simulink model "geometric_control_ceil_ground"  (R2025a)
settings: Solver=VariableStepAuto  StartTime=0.0  StopTime=t_total(end)  RelTol=1e-3
StopFcn:
  | autoplot;
values from neighbouring files (symbols this model uses):
  Ib = diag([params.Ix, params.Iy, params.Iz])    [setup_mission.m]
  lin_vel_0 = [0; 0; 0]    [setup_mission.m]
  mass = params.m    [setup_mission.m]
  pos_0 = p_ref(:,1) + offset_init    [setup_mission.m]
  Ts = dt    (= 0.001)    [setup_mission.m]
  w_bb_0 = [0; 0; 0]    [setup_mission.m]
undefined symbols (not defined in the file or in its folder): dspblkCoreblockFVToolHelper, gcbh
libraries: robotcorelib x2, uavutilslib x1
settings Model: Creator=fabioruggiero  LastModifiedBy=marco
settings ModelReferenceCC: EnableRefExpFcnMdlSchedulingChecks=on
settings RTWCC: GPUComputeCapability=3.5

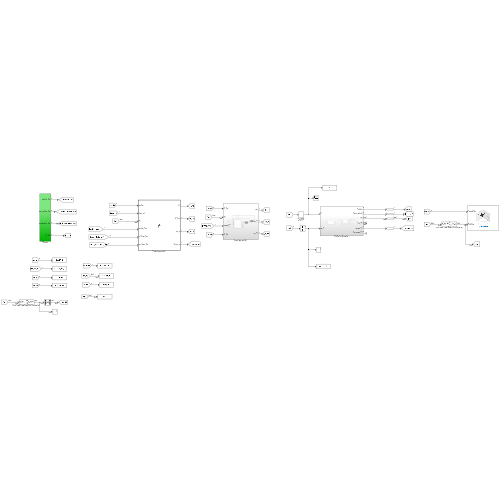
[thumbnail: Simulink's stored preview of the top-level diagram]
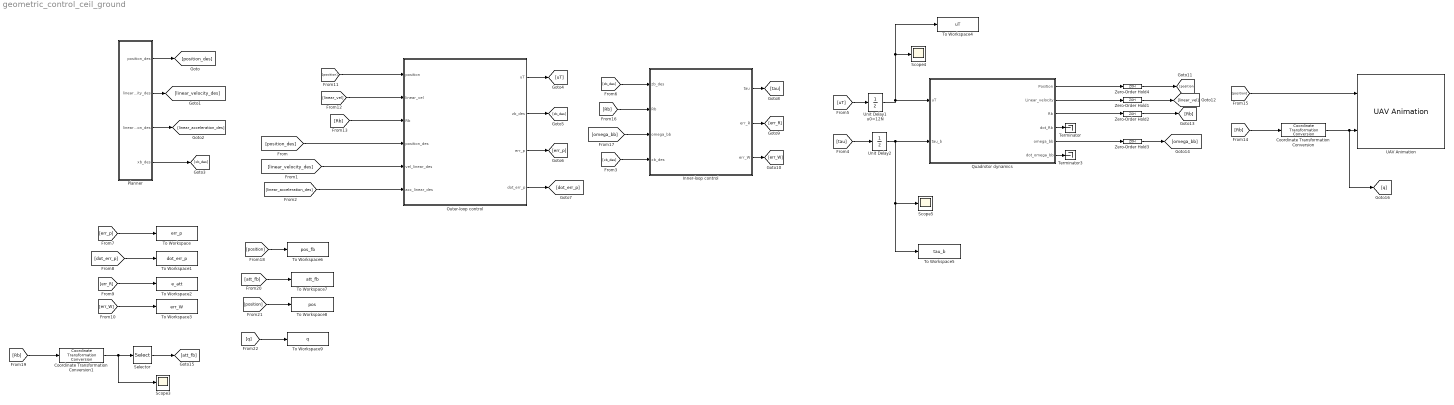
== system geometric_control_ceil_ground ==
  Coordinate Transformation Conversion : robotcorelib/Coordinate Transformation Conversion  InputRepresentation=Rotation Matrix  InputEulerSequence=ZYX  ShowTrVecInputPort=on  OutputRepresentation=Quaternion  OutputEulerSequence=ZYX  ShowTrVecOutputPort=on  SimulateUsing=Interpreted execution
  Coordinate Transformation Conversion1 : robotcorelib/Coordinate Transformation Conversion  InputRepresentation=Rotation Matrix  InputEulerSequence=ZYX  ShowTrVecInputPort=on  OutputRepresentation=Euler Angles  OutputEulerSequence=ZYX  ShowTrVecOutputPort=on  SimulateUsing=Interpreted execution
  Inner-loop control : Subsystem
  Outer-loop control : MATLAB Function  TreatAsAtomicUnit=on
  Planner : Subsystem
  Quadrotor dynamics : Subsystem
  Scope3 : Scope
      settings: ActiveDisplayYMinimum=-1  ActiveDisplayYMaximum=1  DataLoggingVariableName=ScopeData3
  Scope4 : Scope
      settings: ActiveDisplayYMinimum=-1  ActiveDisplayYMaximum=1  DataLoggingVariableName=ScopeData4
  Scope5 : Scope
      settings: ActiveDisplayYMinimum=-1  ActiveDisplayYMaximum=1  DataLoggingVariableName=ScopeData5
  Selector : Selector  InputPortWidth=3  IndexOptions=Index vector (dialog)  Indices=[3, 2, 1]  OutputSizes=1
  Terminator : Terminator
  Terminator3 : Terminator
  To Workspace : ToWorkspace  VariableName=err_p  SaveFormat=Timeseries  SampleTime=Ts
  To Workspace1 : ToWorkspace  VariableName=dot_err_p  SaveFormat=Timeseries  SampleTime=Ts
  To Workspace2 : ToWorkspace  VariableName=e_att  SaveFormat=Timeseries  SampleTime=-1
  To Workspace3 : ToWorkspace  VariableName=err_W  SaveFormat=Timeseries  SampleTime=-1
  To Workspace4 : ToWorkspace  VariableName=uT  SaveFormat=Timeseries  SampleTime=-1
  To Workspace5 : ToWorkspace  VariableName=tau_b  SaveFormat=Timeseries  SampleTime=-1
  To Workspace6 : ToWorkspace  VariableName=pos_fb  SaveFormat=Timeseries  SampleTime=-1
  To Workspace7 : ToWorkspace  VariableName=att_fb  SaveFormat=Timeseries  SampleTime=-1
  To Workspace8 : ToWorkspace  VariableName=pos  SaveFormat=Timeseries  SampleTime=-1
  To Workspace9 : ToWorkspace  VariableName=q  SaveFormat=Timeseries  SampleTime=-1
  UAV Animation : uavutilslib/UAV Animation  NumUAV=1  DynamicUAVConfig=off  UAVType=Multirotor  UAVSize=1  UAVColor=[1 0 0]  UAVTrajectoryAlpha=1  InertialZDirection=Down  RotationFormat=Quaternion  DrawMarkers=off  SampleTime=0.01
  Unit Delay1 u0=12N : UnitDelay  InitialCondition=12  SampleTime=Ts
  Unit Delay2 : UnitDelay  InitialCondition=[0 0 0]  SampleTime=Ts
  Zero-Order Hold{1..4} (4 alike) : ZeroOrderHold  SampleTime=Ts
  wires:
  Unit Delay1 u0=12N/1 -> Quadrotor dynamics/1(uT), To Workspace4/1, Scope4/1
  Quadrotor dynamics/1(Position) -> Zero-Order Hold4/1
  Quadrotor dynamics/2(Linear_velocity) -> Zero-Order Hold1/1
  Quadrotor dynamics/3(Rb) -> Zero-Order Hold2/1
  Quadrotor dynamics/5(omega_bb) -> Zero-Order Hold3/1
  Unit Delay2/1 -> Quadrotor dynamics/2(tau_b), Scope5/1, To Workspace5/1
  Quadrotor dynamics/4(dot_Rb) -> Terminator/1
  Quadrotor dynamics/6(dot_omega_bb) -> Terminator3/1
  Coordinate Transformation Conversion/1 -> [q], UAV Animation/2
  Inner-loop control/2(err_R) -> [err_R]
  Inner-loop control/3(err_W) -> [err_W]
  Planner/1(position_des) -> [position_des]
  Planner/2(linear_velocity_des) -> [linear_velocity_des]
  Planner/3(linear_acceleration_des) -> [linear_acceleration_des]
  Planner/4(xb_des) -> [xb_des]
  [position_des] -> Outer-loop control/4(position_des)
  [linear_velocity_des] -> Outer-loop control/5(vel_linear_des)
  [linear_acceleration_des] -> Outer-loop control/6(acc_linear_des)
  [xb_des] -> Inner-loop control/4(xb_des)
  Outer-loop control/4(dot_err_p) -> [dot_err_p]
  Outer-loop control/3(err_p) -> [err_p]
  Outer-loop control/2(zb_des) -> [zb_des]
  Outer-loop control/1(uT) -> [uT]
  Inner-loop control/1(tau) -> [tau]
  [tau] -> Unit Delay2/1
  [uT] -> Unit Delay1 u0=12N/1
  [zb_des] -> Inner-loop control/1(zb_des)
  [dot_err_p] -> To Workspace1/1
  [err_p] -> To Workspace/1
  [err_R] -> To Workspace2/1
  [err_W] -> To Workspace3/1
  [position] -> Outer-loop control/1(position)
  Zero-Order Hold4/1 -> [position]
  Zero-Order Hold1/1 -> [linear_vel]
  Zero-Order Hold2/1 -> [Rb]
  [Rb] -> Coordinate Transformation Conversion/1
  [position] -> UAV Animation/1
  Zero-Order Hold3/1 -> [omega_bb]
  [Rb] -> Inner-loop control/2(Rb)
  [omega_bb] -> Inner-loop control/3(omega_bb)
  [linear_vel] -> Outer-loop control/2(linear_vel)
  [Rb] -> Outer-loop control/3(Rb)
  [position] -> To Workspace6/1
  Selector/1 -> [att_fb]
  Coordinate Transformation Conversion1/1 -> Selector/1, Scope3/1
  [Rb] -> Coordinate Transformation Conversion1/1
  [att_fb] -> To Workspace7/1
  [position] -> To Workspace8/1
  [q] -> To Workspace9/1

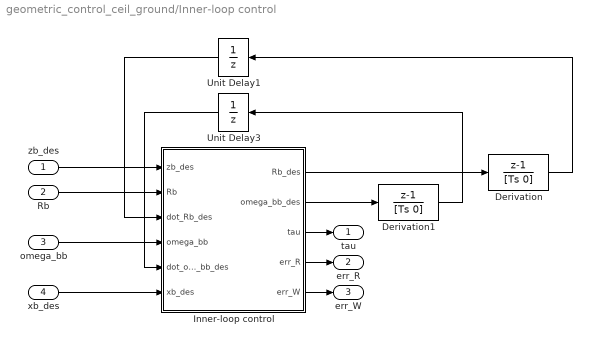
== system geometric_control_ceil_ground/Inner-loop control ==
  zb_des : Inport
  Rb : Inport  Port=2
  omega_bb : Inport  Port=3
  xb_des : Inport  Port=4
  Derivation : DiscreteTransferFcn  Numerator=[1 -1]  Denominator=[Ts 0]  InitialStates=[1 0 0;0 1 0;0 0 1]  SampleTime=Ts
  Derivation1 : DiscreteTransferFcn  LoadFcn=dspblkCoreblockFVToolHelper(gcbh,'load');  Numerator=[1 -1]  Denominator=[Ts 0]  InitialStates=[0 0 0]  SampleTime=Ts
      settings: CopyFcn=dspblkCoreblockFVToolHelper(gcbh,'copy');  DeleteFcn=dspblkCoreblockFVToolHelper(gcbh,'close');  ModelCloseFcn=dspblkCoreblockFVToolHelper(gcbh,'close');  PreSaveFcn=dspblkCoreblockFVToolHelper(gcbh,'presave');  PostSaveFcn=dspblkCoreblockFVToolHelper(gcbh,'postsave');  CloseFcn=dspblkCoreblockFVToolHelper(gcbh,'close');
  Inner-loop control : MATLAB Function  TreatAsAtomicUnit=on
  Unit Delay1 : UnitDelay  InitialCondition=eye(3)  SampleTime=Ts
  Unit Delay3 : UnitDelay  InitialCondition=[0 0 0]  SampleTime=Ts
  tau : Outport
  err_R : Outport  Port=2
  err_W : Outport  Port=3
  wires:
  xb_des/1 -> Inner-loop control/6(xb_des)
  Inner-loop control/4(err_R) -> err_R/1
  Rb/1 -> Inner-loop control/2(Rb)
  Inner-loop control/3(tau) -> tau/1
  Unit Delay1/1 -> Inner-loop control/3(dot_Rb_des)
  Derivation1/1 -> Unit Delay3/1
  Inner-loop control/5(err_W) -> err_W/1
  Unit Delay3/1 -> Inner-loop control/5(dot_omega_bb_des)
  Derivation/1 -> Unit Delay1/1
  zb_des/1 -> Inner-loop control/1(zb_des)
  omega_bb/1 -> Inner-loop control/4(omega_bb)
  Inner-loop control/1(Rb_des) -> Derivation/1
  Inner-loop control/2(omega_bb_des) -> Derivation1/1

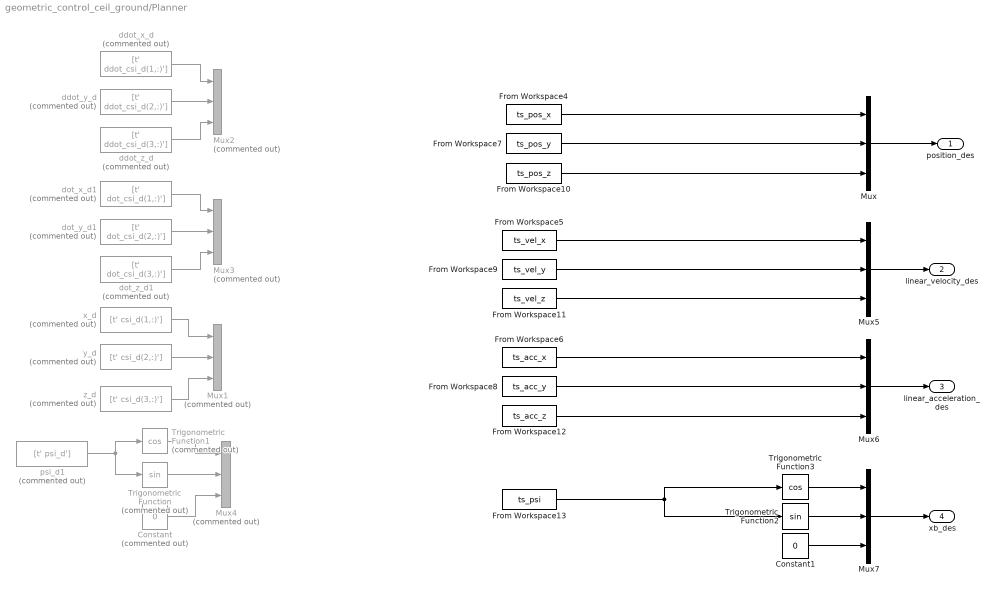
== system geometric_control_ceil_ground/Planner ==
  Constant : Constant  Commented=on  Value=0
  Constant1 : Constant  Value=0
  From Workspace10 : FromWorkspace  VariableName=ts_pos_z
  From Workspace11 : FromWorkspace  VariableName=ts_vel_z
  From Workspace12 : FromWorkspace  VariableName=ts_acc_z
  From Workspace13 : FromWorkspace  VariableName=ts_psi
  From Workspace4 : FromWorkspace  VariableName=ts_pos_x
  From Workspace5 : FromWorkspace  VariableName=ts_vel_x
  From Workspace6 : FromWorkspace  VariableName=ts_acc_x
  From Workspace7 : FromWorkspace  VariableName=ts_pos_y
  From Workspace8 : FromWorkspace  VariableName=ts_acc_y
  From Workspace9 : FromWorkspace  VariableName=ts_vel_y
  Mux{,5..7} (4 alike) : Mux  Inputs=3
  Mux{1..4} (4 alike) : Mux  Commented=on  Inputs=3
  Trigonometric Function : Trigonometry  Commented=on
  Trigonometric Function1 : Trigonometry  Commented=on  Operator=cos
  Trigonometric Function2 : Trigonometry
  Trigonometric Function3 : Trigonometry  Operator=cos
  ddot_x_d : FromWorkspace  Commented=on  VariableName=[t' ddot_csi_d(1,:)']  SampleTime=Ts
  ddot_y_d : FromWorkspace  Commented=on  VariableName=[t' ddot_csi_d(2,:)']  SampleTime=Ts
  ddot_z_d : FromWorkspace  Commented=on  VariableName=[t' ddot_csi_d(3,:)']  SampleTime=Ts
  dot_x_d1 : FromWorkspace  Commented=on  VariableName=[t' dot_csi_d(1,:)']  SampleTime=Ts
  dot_y_d1 : FromWorkspace  Commented=on  VariableName=[t' dot_csi_d(2,:)']  SampleTime=Ts
  dot_z_d1 : FromWorkspace  Commented=on  VariableName=[t' dot_csi_d(3,:)']  SampleTime=Ts
  psi_d1 : FromWorkspace  Commented=on  VariableName=[t' psi_d']  SampleTime=Ts
  x_d : FromWorkspace  Commented=on  VariableName=[t' csi_d(1,:)']  SampleTime=Ts
  y_d : FromWorkspace  Commented=on  VariableName=[t' csi_d(2,:)']  SampleTime=Ts
  z_d : FromWorkspace  Commented=on  VariableName=[t' csi_d(3,:)']  SampleTime=Ts
  position_des : Outport
  linear_velocity_des : Outport  Port=2
  linear_acceleration_des : Outport  Port=3
  xb_des : Outport  Port=4
  wires:
  y_d/1 -> Mux1/2
  z_d/1 -> Mux1/3
  x_d/1 -> Mux1/1
  ddot_y_d/1 -> Mux2/2
  ddot_z_d/1 -> Mux2/3
  ddot_x_d/1 -> Mux2/1
  dot_y_d1/1 -> Mux3/2
  dot_z_d1/1 -> Mux3/3
  dot_x_d1/1 -> Mux3/1
  Trigonometric Function/1 -> Mux4/2
  psi_d1/1 -> Trigonometric Function/1, Trigonometric Function1/1
  Trigonometric Function1/1 -> Mux4/1
  Constant/1 -> Mux4/3
  From Workspace5/1 -> Mux5/1
  From Workspace9/1 -> Mux5/2
  From Workspace11/1 -> Mux5/3
  From Workspace10/1 -> Mux/3
  From Workspace12/1 -> Mux6/3
  From Workspace8/1 -> Mux6/2
  From Workspace7/1 -> Mux/2
  From Workspace4/1 -> Mux/1
  From Workspace6/1 -> Mux6/1
  Mux/1 -> position_des/1
  Mux5/1 -> linear_velocity_des/1
  Mux6/1 -> linear_acceleration_des/1
  Trigonometric Function3/1 -> Mux7/1
  Constant1/1 -> Mux7/3
  Trigonometric Function2/1 -> Mux7/2
  From Workspace13/1 -> Trigonometric Function2/1, Trigonometric Function3/1
  Mux7/1 -> xb_des/1

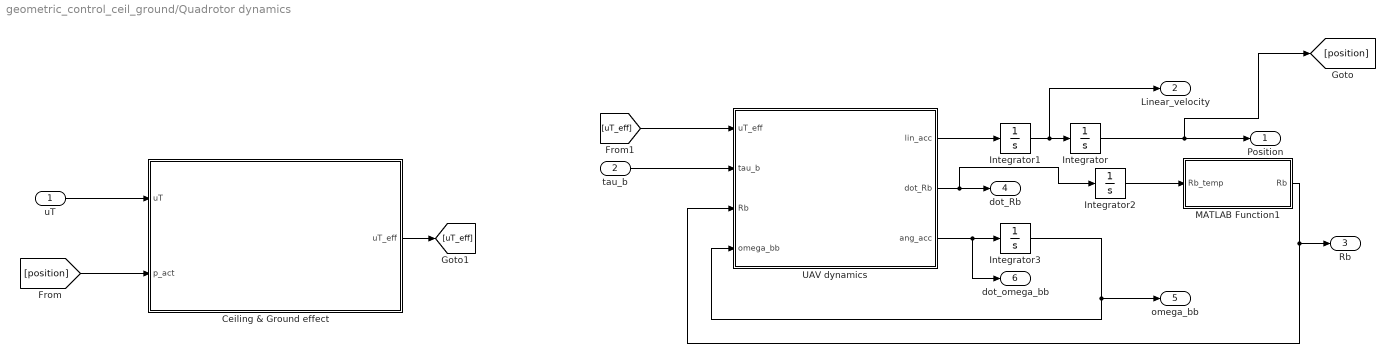
== system geometric_control_ceil_ground/Quadrotor dynamics ==
  uT : Inport
  tau_b : Inport  Port=2
  Ceiling & Ground effect : MATLAB Function  TreatAsAtomicUnit=on
  Integrator : Integrator  InitialCondition=pos_0
  Integrator1 : Integrator  InitialCondition=lin_vel_0
  Integrator2 : Integrator  InitialCondition=[1 0 0; 0 1 0;0 0 1]
  Integrator3 : Integrator  InitialCondition=w_bb_0
  MATLAB Function1 : MATLAB Function  TreatAsAtomicUnit=on
  UAV dynamics : MATLAB Function  TreatAsAtomicUnit=on
  Position : Outport
  Linear_velocity : Outport  Port=2
  Rb : Outport  Port=3
  dot_Rb : Outport  Port=4
  omega_bb : Outport  Port=5
  dot_omega_bb : Outport  Port=6
  wires:
  MATLAB Function1/1(Rb) -> Rb/1, UAV dynamics/3(Rb)
  [uT_eff] -> UAV dynamics/1(uT_eff)
  Integrator1/1 -> Linear_velocity/1, Integrator/1
  [position] -> Ceiling & Ground effect/2(p_act)
  Integrator/1 -> [position], Position/1
  uT/1 -> Ceiling & Ground effect/1(uT)
  UAV dynamics/3(ang_acc) -> dot_omega_bb/1, Integrator3/1
  UAV dynamics/2(dot_Rb) -> Integrator2/1, dot_Rb/1
  Integrator3/1 -> UAV dynamics/4(omega_bb), omega_bb/1
  UAV dynamics/1(lin_acc) -> Integrator1/1
  tau_b/1 -> UAV dynamics/2(tau_b)
  Ceiling & Ground effect/1(uT_eff) -> [uT_eff]
  Integrator2/1 -> MATLAB Function1/1(Rb_temp)

== matlab function geometric_control_ceil_ground/Quadrotor dynamics/Ceiling & Ground effect ==
  data: uT input; uT_eff output; p_act input
function uT_eff = aero_disturbances(uT, p_act)

% --- ENVIRONMENTAL AND DRONE PARAMETERS ---
R = 0.15;           % Propeller radius [m] (Typical OS4)
H_room = 3.0;       % Room height [m] 

% Ceiling Effect Coefficients
k1 = 6.924;
k2 = 0.03782;

% --- DISTANCES CALCULATION  ---
z_drone = p_act(3);         % Current altitude (negative in flight)
d_ground = -z_drone;        % Distance from floor (z=0)
d_ceil   = H_room - d_ground; % Distance from ceiling (z=-3)

% Safety saturation to prevent division by zero
d_ground = max(0.05, d_ground);
d_ceil   = max(0.05, d_ceil);

% --- GROUND EFFECT ---
K_ground = 1.0;
if d_ground < (2 * R)
    ratio_g = (R / (4 * d_ground))^2;
    ratio_g = min(ratio_g, 0.9); % Saturation to prevent singularities
    K_ground = 1 / (1 - ratio_g);
end

% --- CEILING EFFECT ---
K_ceil = 1.0;
if d_ceil < (2 * R)
    term_num = (R / (d_ceil + k2))^2;
    term_den = k1;
    ratio_c  = term_num / term_den;
    ratio_c  = min(ratio_c, 0.9); % Saturation
    K_ceil   = 1 / (1 - ratio_c);
end
% --- EFFECTIVE THRUST CALCULATION ---
K_tot = K_ground * K_ceil;
uT_eff = uT * K_tot;
end

== matlab function geometric_control_ceil_ground/Quadrotor dynamics/UAV dynamics ==
  data: uT_eff input size=1; tau_b input size=3; lin_acc output size=3; Rb input size=[3,3]; omega_bb input size=3; dot_Rb output size=[3,3]; ang_acc output size=3; mass parameter size=1; Ib parameter size=[3,3]
function [lin_acc, dot_Rb, ang_acc] = uav_dynamics(uT_eff, tau_b, Rb, omega_bb, mass, Ib)

% --- PARAMETRIC UNCERTAINTY ---

m_real = mass * 1.4; 
g = 9.81;
e3 = [0; 0; 1];

% --- TRANSLATIONAL DYNAMICS ---

Thrust_Inertial = (uT_eff / m_real) * Rb * e3;

lin_acc = g * e3 - Thrust_Inertial; 

% --- ROTATIONAL DYNAMICS ---
dot_Rb = Rb * skew(omega_bb);
ang_acc = Ib \ (-skew(omega_bb) * Ib * omega_bb + tau_b);
end
function S = skew(v)
if(numel(v)~= 1)
    S= [0 -v(3) v(2); v(3) 0 -v(1); -v(2) v(1) 0];
else
    S= zeros(3);
end
end

== matlab function geometric_control_ceil_ground/Outer-loop control ==
  data: position input size=3; uT output size=1; linear_vel input size=3; Rb input size=[3,3]; zb_des output size=3; mass parameter size=1; position_des input size=3; vel_linear_des input size=3; acc_linear_des input size=3; err_p output size=3; dot_err_p output size=3
function [uT, zb_des, err_p, dot_err_p] = fcn(position, linear_vel, Rb, mass, ...
    position_des, vel_linear_des, acc_linear_des)
%% OUTER-LOOP CONTROL (MODEL MISMATCH - PURE)
% Versione senza protezioni numeriche.
% Usa forzatamente la massa nominale per evidenziare il difetto di robustezza.

% --- 1. PARAMETRI MODELLO (Fissi per il mismatch) ---
mass_model = 0.468; % Il controllore crede di essere leggero

g = 9.81;
e_3 = [0; 0; 1];

% --- 2. GUADAGNI (TUNING) ---
k_px = 2;   k_py = 2;   k_pz = 5;
k_vx = 1.5; k_vy = 1.5; k_vz = 3;

K_p = diag([k_px, k_py, k_pz]);
K_v = diag([k_vx, k_vy, k_vz]);

% --- 3. CALCOLO ERRORI ---
err_p = position - position_des;
dot_err_p = linear_vel - vel_linear_des;

% --- 4. LEGGE DI CONTROLLO GEOMETRICA ---
% Forza desiderata in coordinate inerziali (Feedforward + Feedback PD)
% Nota: usa mass_model, non mass!
F_des = -K_p*err_p - K_v*dot_err_p - mass_model*g*e_3 + mass_model*acc_linear_des;

% Direzione dell'asse Z del body desiderata (Normalizzazione pura)
% Assumiamo che norm(F_des) > 0 sempre.
zb_des = -F_des / norm(F_des);

% Spinta Totale (Proiezione su Z body attuale)
uT = -F_des' * Rb * e_3;

end

== matlab function geometric_control_ceil_ground/Inner-loop control/Inner-loop control ==
  data: Rb_des output size=[3,3]; omega_bb_des output size=3; tau output size=3; zb_des input size=3; Rb input size=[3,3]; dot_Rb_des input size=[3,3]; omega_bb input size=3; dot_omega_bb_des input size=3; xb_des input size=3; Ib parameter size=[3,3]; err_R output size=3; err_W output size=3
function [Rb_des,omega_bb_des,tau,err_R,err_W] = fcn(zb_des,Rb,dot_Rb_des,omega_bb,dot_omega_bb_des,xb_des,Ib)

%% WRITE HERE THE INNER-LOOP CONTROL
% zb_des: desired z-axis of the body frame
% Rb: current rotation matrix
% dot_Rb_des: time-derivative of the desired rotation matrix
% omega_bb: current angular velocity expressed in the body frame
% dot_omega_bb_des: desired angular acceleration expressed in the body
% frame
% xb_des: desired x-axis of the body frame form the planner
% Ib: inertia matrix of the UAV with respect to the body frame
% ---
% Rb_des: desired rotation matrix
% omega_bb_des: desired angular velocity expressed in the body frame (given
% below as a hint)
% tau: commanded control torque
% err_R: rotational error in SO(3)
% err_W: angular velocity error in SO(3)

k_rx = 10;
k_ry = 10;
k_rz = 5;

k_wx = 1;
k_wy = 1;
k_wz = 1;

K_r = diag([k_rx, k_ry, k_rz]);
K_w = diag([k_wx, k_wy, k_wz]);

%K_r = 15*eye(3);
%K_w = 15*eye(3);

yb_des = (skew(zb_des)*xb_des)/norm(skew(zb_des)*xb_des);

Rb_des = [skew(yb_des)*zb_des, yb_des, zb_des];

omega_bb_des = wedge(Rb_des'*dot_Rb_des);

err_R = 0.5*wedge(Rb_des'*Rb - Rb'*Rb_des);

err_W = omega_bb - Rb'*Rb_des*omega_bb_des;

tau = -K_r*err_R - K_w*err_W + skew(omega_bb)*Ib*omega_bb - Ib*(skew(omega_bb)*Rb'*Rb_des*omega_bb_des-Rb'*Rb_des*dot_omega_bb_des); 

end

function S = skew(v)
if(numel(v)~= 1)
S= [0 -v(3) v(2); 
    v(3) 0 -v(1);
    -v(2) v(1) 0];
else
S= zeros(3);
end
end

function v = wedge(S)
v1 = S(3,2);
v2 = S(1,3);
v3 = S(2,1);
v = [v1 v2 v3]';
end

== matlab function geometric_control_ceil_ground/Quadrotor dynamics/MATLAB Function1 ==
  data: Rb_temp input; Rb output
function Rb = fcn(Rb_temp)
    [U,S,V] = svd(Rb_temp);
    sigma = det(U*V');
    S_ = diag([1 1 sigma]);

    Rb = U*S_*V';
end
